simulink model "untitled"  (R2023a)
settings: Solver=VariableStepAuto  StartTime=0.0  StopTime=10.0  RelTol=1e-3
settings Model: Creator=romav  LastModifiedBy=romav

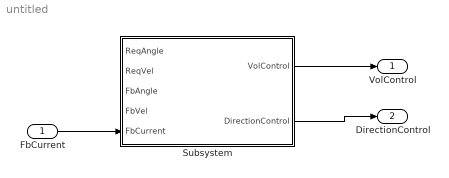
== system untitled ==
  FbCurrent : Inport
  Subsystem : Subsystem
  VolControl : Outport
  DirectionControl : Outport  Port=2
  wires:
  FbCurrent/1 -> Subsystem/5(FbCurrent)
  Subsystem/1(VolControl) -> VolControl/1
  Subsystem/2(DirectionControl) -> DirectionControl/1

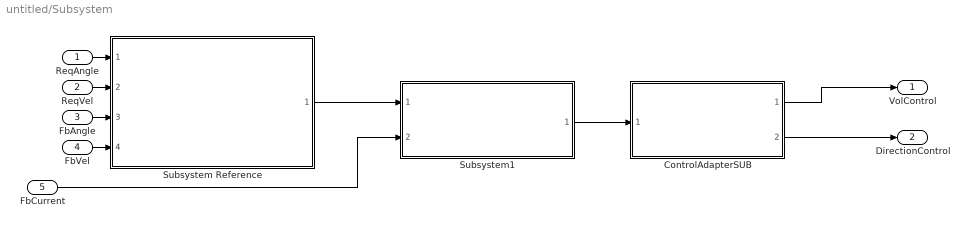
== system untitled/Subsystem ==
  ReqAngle : Inport
  ReqVel : Inport  Port=2
  FbAngle : Inport  Port=3
  FbVel : Inport  Port=4
  FbCurrent : Inport  Port=5
  ControlAdapterSUB : Subsystem  ReferencedSubsystem=ControlAdapterSUB
  Subsystem Reference : Subsystem  ReferencedSubsystem=HighLevelControlSUB
  Subsystem1 : Subsystem  ReferencedSubsystem=LowLevelControllerSUB
  VolControl : Outport
  DirectionControl : Outport  Port=2
  wires:
  ReqAngle/1 -> Subsystem Reference/1
  FbAngle/1 -> Subsystem Reference/3
  ReqVel/1 -> Subsystem Reference/2
  Subsystem1/1 -> ControlAdapterSUB/1
  Subsystem Reference/1 -> Subsystem1/1
  FbVel/1 -> Subsystem Reference/4
  ControlAdapterSUB/1 -> VolControl/1
  FbCurrent/1 -> Subsystem1/2
  ControlAdapterSUB/2 -> DirectionControl/1
